simulink subsystem "MultiShapeOscillator"  (R2024a)
settings: Solver=VariableStepAuto  StartTime=0.0  StopTime=10.0  RelTol=1e-3
undefined symbols (not defined in the file or in its folder): vmax, vmin, wave_len
settings Model: Creator=dfurodet  LastModifiedBy=david

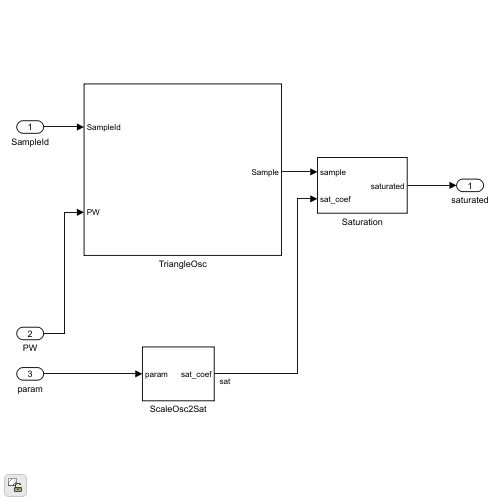
[thumbnail: Simulink's stored preview of the top-level diagram]
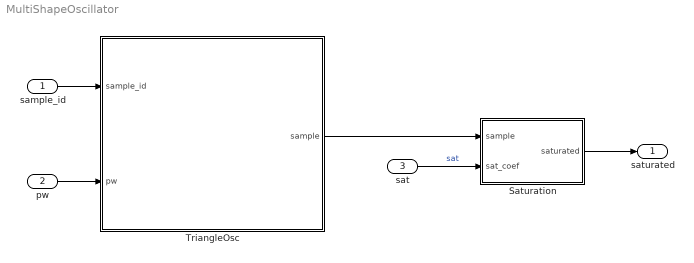
== system MultiShapeOscillator ==
  sample_id : Inport
  pw : Inport  Port=2
  sat : Inport  Port=3
  Saturation : Subsystem
  TriangleOsc : Subsystem  Description=|
      | Oscillator that produces a triangle signal with a given pulse width
      | 
      | A null pulse width results in an inverted sawtooth, a pulse width greater or equal to the wave length produces a sawtooth.
      | The signals in between are variations of a triangle signal.
  saturated : Outport
  wires:
  TriangleOsc/1(sample) -> Saturation/1(sample)
  sat/1 -> Saturation/2(sat_coef)  "sat"
  pw/1 -> TriangleOsc/2(pw)
  Saturation/1(saturated) -> saturated/1
  sample_id/1 -> TriangleOsc/1(sample_id)

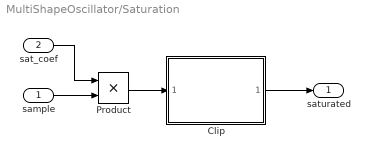
== system MultiShapeOscillator/Saturation ==
  sample : Inport
  sat_coef : Inport  Port=2
  Clip : Subsystem  ReferencedSubsystem=Clip
  Product : Product
  saturated : Outport
  wires:
  Clip/1 -> saturated/1
  Product/1 -> Clip/1
  sat_coef/1 -> Product/1
  sample/1 -> Product/2

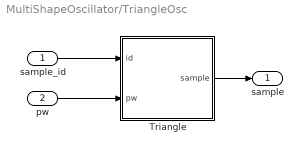
== system MultiShapeOscillator/TriangleOsc ==
  sample_id : Inport
  pw : Inport  Port=2
  Triangle : MATLAB Function  TreatAsAtomicUnit=on
  sample : Outport
  wires:
  pw/1 -> Triangle/2(pw)
  Triangle/1(sample) -> sample/1
  sample_id/1 -> Triangle/1(id)

== matlab function MultiShapeOscillator/TriangleOsc/Triangle ==
  data: id input; sample output; pw input; wave_len parameter; vmin parameter; vmax parameter
function sample = triangle_signal(id, pw, wave_len, vmin, vmax)
amp = vmax - vmin;
if id < pw
    sample = vmin + amp * id / pw;
else
    slope = wave_len - pw;
    sample = vmax - amp * (id - pw) / slope;
end
